simulink model "TwoLegRobotSim"  (R2022b)
settings: Solver=VariableStepAuto  StartTime=0.0  StopTime=20  MaxStep=1e-4  MinStep=1e-6  RelTol=1e-3
model workspace: external: MATLAB File D:\5720\Tutorial 2\TwoLegRobot_DataFile.m (data not in the file)
undefined symbols (not defined in the file): base_params, current_params, k_cols, k_rows, Mass_body, Mass_lower_leg, Mass_upper_leg, Mass_wheel, P0, p_matrix, qphi, qth, qx, R_k, smiData, X, X0_hat, Y, Z
libraries: sm_lib x79, nesl_utility x17, slpidlib x5
(part 4 of 4)

== matlab function TwoLegRobotSim/MATLAB Function ==
  settings: updateMethod=DISCRETE
  data: X_hat_out output; current_input input; dt input; Zk input; R_k parameter; base_params parameter; L input; qx parameter; qth parameter; qphi parameter; reset input; X0_hat parameter; P0 parameter; est_out output
function [X_hat_out, est_out]  = ekf_observer_mem( ...
    current_input, dt, Zk, R_k, base_params, L, qx, qth, qphi, ...
    reset, X0_hat, P0)
%#codegen
persistent P_bk_int
persistent current_state_inner
if isempty(P_bk_int) || reset
    P_bk_int = P0;                 % seed covariance here
end

if isempty(current_state_inner) || reset
    current_state_inner = X0_hat;                 % seed covariance here
end

if isempty(current_input) || reset
    current_input = [0;0];                 % no control provided
end


% Call your existing one-step EKF (returns posterior)
[X_hat_out, P_out,est_out] = ekf_observer( ...
    current_state_inner, current_input, dt, Zk, R_k, base_params, L, qx, qth, qphi, P_bk_int);

% Store posterior as next prior
P_bk_int = P_out;
current_state_inner = X_hat_out;
end





function [X_k_hat_f,Pk_f,X_k_hat] = ekf_observer( ...
    current_state, current_input, dt, Zk, R_k,base_params, L,qx, qth, qphi, P_bk)
%#codegen
% EKF observer step (predict -> linearize -> cov predict -> update).
% Sizes:
%   current_state : 6x1  [x; dx; theta; dtheta; phi; dphi]
%   current_input : ?x1  (your actuator vector)
%   dt            : 1x1
%   Zk            : 3x1  [dx; theta; phi]
%   R_k           : 3x3
%   Q_k           : 6x6  (DISCRETE process noise)
%   P_bk          : 6x6  (prior covariance)
%   base_params: struct with fields used below
%
% Outputs:
%   X_k_hat_f : 6x1  (posterior state)
%   Pk_f      : 6x6  (posterior covariance)
%   X_k_hat   : 6x1  (prior/predicted state)
%   Pk        : 6x6  (prior/predicted covariance)
%   K_f       : 6x3  (Kalman gain)
%   S         : 3x3  (innovation covariance)

% -------- 1) Nonlinear prediction (explicit Euler, consistent with Fk = I + dt*A) --------

Q_k = make_Q(dt, qx, qth, qphi);

[inertia_val, l_num, l_m_num] = inertia_calculator(L);

acc = accel_func_generated( ...
    current_state, ...
    current_input, ...
    base_params.M, ...
    base_params.mp, ...
    base_params.IM, ...
    inertia_val,...
    base_params.l, ...
    l_num, ...
    l_m_num, ...
    base_params.R, ...
    base_params.g, ...
    base_params.m_w, ...
    base_params.I_wheel );

ddx     = acc(1);
ddtheta = acc(2);
ddphi   = acc(3);

% velocities (one-step integration of accelerations)
dx_pred     = current_state(2) + dt * ddx;
dtheta_pred = current_state(4) + dt * ddtheta;
dphi_pred   = current_state(6) + dt * ddphi;

% positions/angles (explicit Euler with old velocities — matches Fk choice)
x_pred     = current_state(1) + dt * current_state(2);
theta_pred = current_state(3) + dt * current_state(4);
phi_pred   = current_state(5) + dt * current_state(6);

% prior state
X_k_hat = [x_pred; dx_pred; theta_pred; dtheta_pred; phi_pred; dphi_pred];

% optional: wrap angles in the state (keeps them bounded)
X_k_hat(3) = atan2(sin(X_k_hat(3)), cos(X_k_hat(3)));
X_k_hat(5) = atan2(sin(X_k_hat(5)), cos(X_k_hat(5)));

% -------- 2) Linearization (continuous-time Jacobian) --------
A_c = jacobian_Ac_generated( ...
    current_state, ...
    current_input, ...
    base_params.M, ...
    base_params.mp, ...
    base_params.IM, ...
    inertia_val,...
    base_params.l, ...
    l_num, ...
    l_m_num, ...
    base_params.R, ...
    base_params.g, ...
    base_params.m_w, ...
    base_params.I_wheel );

% -------- 3) Discretization consistent with Euler state step --------
Fk = eye(6) + dt * A_c;

% -------- 4) Covariance predict --------
Pk = Fk * P_bk * Fk.' + Q_k;
Pk = 0.5 * (Pk + Pk.');  % symmetrize (numerical hygiene)

% -------- 5) Measurement model --------
% Measures [dx; theta; phi] in that order
H_k = [0,1,0,0,0,0; ...
       0,0,1,0,0,0; ...
       0,0,0,0,1,0];

S   = H_k*Pk*H_k.' + R_k;

% Solve for K without explicit inverse (codegen-friendly)
K_f = (Pk*H_k.') / S;

% -------- 6) Innovation (wrap angle residuals) --------
innov = Zk - H_k*X_k_hat;
% wrap theta, phi residuals to [-pi,pi]
innov(2) = atan2(sin(innov(2)), cos(innov(2)));
innov(3) = atan2(sin(innov(3)), cos(innov(3)));

% -------- 7) State update --------
X_k_hat_f = X_k_hat + K_f * innov;

% wrap updated angles
X_k_hat_f(3) = atan2(sin(X_k_hat_f(3)), cos(X_k_hat_f(3)));
X_k_hat_f(5) = atan2(sin(X_k_hat_f(5)), cos(X_k_hat_f(5)));

% -------- 8) Joseph-form covariance update --------
I6   = eye(6);
Pk_f = (I6 - K_f*H_k) * Pk * (I6 - K_f*H_k).' + K_f * R_k * K_f.';
Pk_f = 0.5 * (Pk_f + Pk_f.');  % symmetrize

end



function [I,LH,LL] = inertia_calculator(L_input)
    %#codegen
    % Solves for theta1, theta2 from:
    %   2*L1*sin(theta1) + 2*L2*sin(theta2) = L_input
    %   0.5*LR + 2*L1*cos(theta1) - 2*L2*cos(theta2) = 0
    % using a few Newton steps (no function handles, codegen-safe).
    
    % Constants (same as your previous function)
    L1 = 0.07;  L2 = 0.105;
    M1 = 0.3;   M2 = 0.3;    % not used directly but retained for clarity
    M3 = 0.5;   M4 = 0.5;
    LR = 0.2;
    
    % Initial guess (could be persisted across calls for faster convergence)
    theta1 = 0.2;
    theta2 = 0.0;
    
    % Newton iterations (small, damped)
    for it = 1:10
        s1 = sin(theta1); c1 = cos(theta1);
        s2 = sin(theta2); c2 = cos(theta2);
    
        f1 = 2*L1*s1 + 2*L2*s2 - L_input;
        f2 = 0.5*LR + 2*L1*c1 - 2*L2*c2;
    
        % Jacobian
        J11 =  2*L1*c1;   J12 =  2*L2*c2;
        J21 = -2*L1*s1;   J22 =  2*L2*s2;
    
        % Solve J * d = -f  (2x2 solve)
        detJ = J11*J22 - J12*J21;
        if abs(detJ) < 1e-12
            break; % singular Jacobian; leave current guess
        end
        d1 = (-f1*J22 + f2*J12)/detJ;
        d2 = (-J11*f2 + J21*f1)/detJ;
    
        % Damping + update
        alpha = 0.7;
        theta1 = theta1 + alpha*d1;
        theta2 = theta2 + alpha*d2;
    
        % Clamp to bounds (your original lb/ub)
        if theta1 < 0,       theta1 = 0;     end
        if theta1 > pi,      theta1 = pi;    end
        if theta2 < -pi/2,   theta2 = -pi/2; end
        if theta2 >  pi/2,   theta2 =  pi/2; end
    
        if (abs(d1)+abs(d2)) < 1e-9
            break;
        end
    end
    
    % Geometry
    I_l = 2827482.39e-9;   % long leg inertia
    I_h = 586653.56e-9;    % short leg inertia
    
    y1 = L1*sin(theta1);
    y3 = 2*y1 + L2*sin(theta2);
    
    % COM split
    LH = (y1*M1 + y1*M2 + y3*M3 + y3*M4) / (M1 + M2 + M3 + M4);
    LL = L_input - LH;
    
    % Distances
    LHR = sqrt((LH - y1)^2 + (LR/2 + L1*cos(theta1))^2);
    LLR = sqrt((y3 - LH)^2 + (L2*cos(theta2))^2);
    
    % Inertia
    I = 2*(I_h + M1*LHR^2) + 2*(I_l + M3*LLR^2);
end


% function Q_k = make_Q(dt, qdx, qth, qphi)
% %make_Q Generates the 6x6 DISCRETE state weighting matrix Q_k for a discrete-time LQR controller.
% %
% %   This function creates the Q matrix for the 6-state wheel-legged robot
% %   model. It does NOT include the augmented state for integral action.
% %
% %   The state vector is assumed to be in the order:
% %   [X, X_dot, theta, theta_dot, phi, phi_dot]
% %
% %   Inputs:
% %       dt          - The sample time (time step) used for discretization.
% %       qdx         - Weight for the forward velocity (X_dot).
% %       qth         - Weight for the leg angle (theta).
% %       qphi        - Weight for the body pitch angle (phi).
% %
% %   Output:
% %       Q_k         - The 6x6 diagonal discrete-time state weighting matrix.
% %
% %   Usage Example:
% %       dt = 0.01;
% %       Q_k = make_Q(dt, 200, 10, 5000);
% 
% % --- Input Validation (Optional but Recommended) ---
% if nargin ~= 4
%     error('make_Q requires exactly 4 input arguments: dt, qdx, qth, qphi');
% end
% 
% % --- Define Continuous-Time Weights for Damping (Velocity Terms) ---
% % The weights for velocity states are set as a fraction of their
% % corresponding position state weights to provide damping.
% q_theta_dot = 0.1 * qth;   % Damping for the leg angle
% q_phi_dot   = 0.1 * qphi;    % Damping for the body pitch
% 
% % --- Define Continuous-Time Weight for Absolute Position ---
% % For a velocity controller, the absolute position is generally not
% % penalized. A very small value is used for numerical stability.
% q_x_pos = 1e-6;
% 
% % --- Assemble the CONTINUOUS 6x6 Diagonal Q Matrix ---
% % First, we define the weights as if for a continuous system.
% % The order of weights must match the state vector order:
% % [X,      X_dot, theta, theta_dot, phi,    phi_dot]
% Q_continuous = diag([q_x_pos, qdx,   qth,   q_theta_dot, qphi,   q_phi_dot]);
% 
% % --- Discretize the Q matrix ---
% % A common method for discretizing the LQR cost function is to scale
% % the continuous state weighting matrix by the sample time dt.
% Q_k = Q_continuous * dt;
% 
% end


function Qk = make_Q(dt, qx, qth, qphi)
%#codegen
dt  = max(dt, eps);
dt2 = dt*dt; dt3 = dt2*dt;
Q2  = @(q) [q*dt3/3, q*dt2/2; q*dt2/2, q*dt];
Qk  = blkdiag(Q2(qx), Q2(qth), Q2(qphi));
Qk  = 0.5*(Qk+Qk.');           % keep symmetric
end

== matlab function TwoLegRobotSim/MATLAB Function5 ==
  data: t_now input; t_prev input; dt output; reset input; Ts_default input
function dt = dttime_stateless(t_now, t_prev, reset, Ts_default)
%#codegen
if reset
    dt = Ts_default;
else
    dt = t_now - t_prev;
    if dt <= 0
        dt = Ts_default;
    end
end
end

== matlab function TwoLegRobotSim/MATLAB Function6 ==
  data: dx input; theta input; Z_k output; phi input
function Z_k   = Mux(dx,theta,phi)
    Z_k = [dx;theta;phi];
end

== matlab function TwoLegRobotSim/MATLAB Function7 ==
  data: theta input; Fn output; dtheta input; ddtheta input; L input; dL input; ddL input; ddZm input; base_params parameter; F input; Tp input
function Fn = fcn(theta,dtheta,ddtheta,L,dL,ddL,ddZm,base_params,F,Tp)
    az = 2*sin(theta)*dL*dtheta - cos(theta)*ddL + ddZm + cos(theta)*L*dtheta^2+sin(theta)*L*ddtheta;
    mw = base_params.m_w/2;
    P = F*cos(theta)+(Tp*sin(theta)/(L));
    Fn = mw*az+P+mw*9.81;

== matlab function TwoLegRobotSim/Fsup ==
  data: u1 input; y output; u2 input
function y = averageTwoInputs(u1,u2)
a = (u1+u2)/2;
if a > 8
    y = 1;
else
    y=0;
end

== matlab function TwoLegRobotSim/dtheta ==
  data: u1 input; y output; u2 input
function y = averageTwoInputs(u1,u2)
y = (u1+u2)/2;

== matlab function TwoLegRobotSim/theta ==
  data: u1 input; y output; u2 input
function y = averageTwoInputs(u1,u2)
y = (u1+u2)/2;

== matlab function TwoLegRobotSim/Subsystem2/MATLAB Function ==
  data: phi1 input; L0 output; phi4 input; phi0 output
function [L0, phi0]  = calculateKinematics(phi1, phi4)
    L1 = 0.14;
    L2 = 0.25;
    L3 = 0.25;
    L4 = 0.14;
    L5 = 0.21;  % between A and E

    % Define coordinates
    XB = -L1*cos(pi-phi1);
    YB = L1*sin(pi-phi1);
    XD = L5+L4*cos(phi4);
    YD = L4*sin(phi4);
    
    A = 2*L2*(XD-XB);
    B = 2*L2*(YD-YB);
    LBD2=(XB-XD)^2+(YB-YD)^2;
    C = L2^2+LBD2-L3^2;

     % Check for reachability
    discriminant = A^2 + B^2 - C^2;
    
    if discriminant < 0
        % This configuration is not reachable
        L0 = 0;
        phi0 = 0;
        return; % Exit the function
    end
    
    % Now it's safe to calculate phi2
    phi2 = 2*atan((B+sqrt(discriminant))/(A+C));
    
    
    % Compute end effector point
    XC = XB + L2*cos(phi2);
    YC = YB + L2*sin(phi2);
    
    
    L0 = sqrt((L5/2 - XC)^2 + YC^2);
    
    if (XC <= (L5/2))
        phi0 = pi - asin(YC / L0) - 0.5*pi;
    else 
        phi0 = asin(YC / L0)-0.5*pi;
    end
end

== matlab function TwoLegRobotSim/Subsystem1/MATLAB Function ==
  data: phi1 input; L0 output; phi4 input; phi0 output
function [L0, phi0]  = calculateKinematics(phi1, phi4)
    L1 = 0.14;
    L2 = 0.25;
    L3 = 0.25;
    L4 = 0.14;
    L5 = 0.21;  % between A and E

    % Define coordinates
    XB = -L1*cos(pi-phi1);
    YB = L1*sin(pi-phi1);
    XD = L5+L4*cos(phi4);
    YD = L4*sin(phi4);
    
    A = 2*L2*(XD-XB);
    B = 2*L2*(YD-YB);
    LBD2=(XB-XD)^2+(YB-YD)^2;
    C = L2^2+LBD2-L3^2;

     % Check for reachability
    discriminant = A^2 + B^2 - C^2;
    
    if discriminant < 0
        % This configuration is not reachable
        L0 = 0;
        phi0 = 0;
        return; % Exit the function
    end
    
    % Now it's safe to calculate phi2
    phi2 = 2*atan((B+sqrt(discriminant))/(A+C));
    
    
    % Compute end effector point
    XC = XB + L2*cos(phi2);
    YC = YB + L2*sin(phi2);
    
    
    L0 = sqrt((L5/2 - XC)^2 + YC^2);
    
    if (XC <= (L5/2))
        phi0 = pi - asin(YC / L0) - 0.5*pi;
    else 
        phi0 = asin(YC / L0)-0.5*pi;
    end
end

== matlab function TwoLegRobotSim/MATLAB Function1 ==
  data: theta input; Fn output; dtheta input; ddtheta input; L input; dL input; ddL input; ddZm input; base_params parameter; F input; Tp input
function Fn = fcn(theta,dtheta,ddtheta,L,dL,ddL,ddZm,base_params,F,Tp)
    az = 2*sin(theta)*dL*dtheta - cos(theta)*ddL + ddZm + cos(theta)*L*dtheta^2+sin(theta)*L*ddtheta;
    mw = base_params.m_w/2;
    P = F*cos(theta)+(Tp*sin(theta)/(L));
    Fn = mw*az+P+mw*9.81;

== matlab function TwoLegRobotSim/MATLAB Function2 ==
  data: u input; T output; Tp output
function [T,Tp]  = Demux(u)
    T = u(1);  % Access the FIRST element
    Tp = u(2); % Access the SECOND element
end

== matlab function TwoLegRobotSim/Matrix Disabler ==
  settings: updateMethod=DISCRETE
  data: u input; out output; sys input; L input; p_matrix parameter; k_rows parameter; k_cols parameter; Ts input; a output
function [out,a]  = fcn(u,sys,L, p_matrix,k_rows, k_cols, Ts)
    persistent xI
    if isempty(xI), xI = 0; end
    %% 4. Use the Fitted Model for Interpolation
    % Suppose we need to calculate the K matrix for a new L value.
    K = zeros(k_rows, k_cols);
    
    % Loop through each element of K that needs to be calculated
    for r = 1:k_rows
        for c = 1:k_cols
            % Calculate the linear index to find the correct row in p_matrix
            idx = (r - 1) * k_cols + c;
            
            % Get the coefficients from the corresponding row
            coefficients = p_matrix(idx, :);
            
            % Use polyval with the coefficients for the current L value
            K(r, c) = polyval(coefficients, L);
        end
    end
    
    % --- The rest of the logic is the same ---
    % Construct the M matrix based on the input u
    M = [u, u, u, u, u, u, u;
         u, u, u, u, u, u, u];
    
    % Perform the run-time calculations
    K_act = M .* K; % Note: Using the dynamically calculated K

    % ---- 3) Velocity-error integrator (track sys(2)) ----
    y_v = sys(2);                   % xdot estimate
    e_v = - y_v;                % velocity error
    % (optional leak: set tau_leak finite to add anti-windup bias bleed)
    xI = xI + Ts*e_v;
    
    % ---- 4) Stack [x; xI] for the 7-state gain ----
    % Expect sys to be 6×1 (plant only). If someone passes 7, ignore their 7th.
    z = [sys(1:6); xI];         % 7×1

    out = -K_act * z;
    a = y_v;
end

== matlab function TwoLegRobotSim/MATLAB Function3 ==
  data: T input; T1 output; T2 output; F input; phi1 input; phi4 input
function [T1,T2] = VMC(T,F,phi1,phi4)
    J = calculateJacobian(phi1,phi4);
    Trob = J'*[F;T];
    T1 = Trob(1);
    T2 = Trob(2);
end
